simulink model "prob1"  (R2020b)
settings: Solver=FixedStepAuto  StartTime=0.0  StopTime=10.0  FixedStep=0.01  RelTol=1e-3
settings Model: Creator=WELCOME  LastModifiedBy=WELCOME

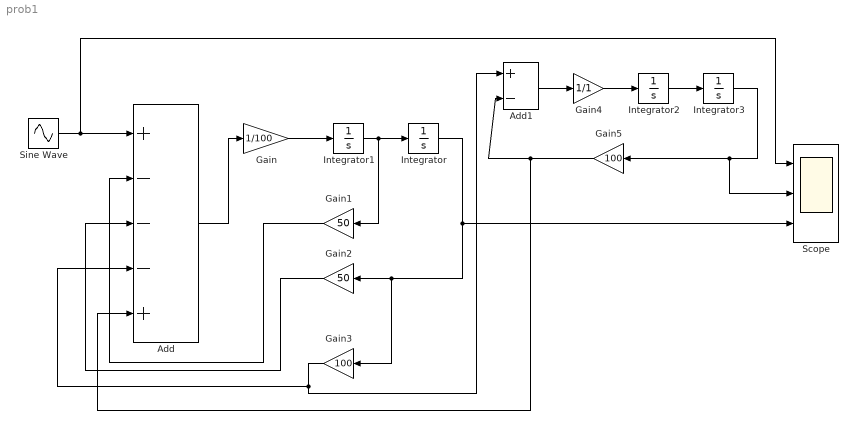
== system prob1 ==
  Add : Sum  Inputs=+---+
  Add1 : Sum  Inputs=+-
  Gain : Gain  Gain=1/100
  Gain1 : Gain  Gain=50
  Gain2 : Gain  Gain=50
  Gain3 : Gain  Gain=100
  Gain4 : Gain  Gain=1/1
  Gain5 : Gain  Gain=100
  Integrator{,1..3} (4 alike) : Integrator
  Scope : Scope  NumInputPorts=3
  Sine Wave : Sin  Amplitude=2  Frequency=10  SampleTime=0
  wires:
  Sine Wave/1 -> Scope/1, Add/1
  Add/1 -> Gain/1
  Integrator1/1 -> Gain1/1, Integrator/1
  Gain/1 -> Integrator1/1
  Gain1/1 -> Add/2
  Gain2/1 -> Add/3
  Integrator/1 -> Scope/3, Gain3/1, Gain2/1
  Gain3/1 -> Add/4, Add1/1
  Add1/1 -> Gain4/1
  Gain4/1 -> Integrator2/1
  Integrator2/1 -> Integrator3/1
  Integrator3/1 -> Scope/2, Gain5/1
  Gain5/1 -> Add/5, Add1/2
